simulink model "FSFB_FF_HIL_quick_dirty"  (R2022a)
settings: Solver=FixedStepAuto  StartTime=tspan(1)  StopTime=tspan(2)  FixedStep=Ts  RelTol=1e-9
undefined symbols (not defined in the file): A, B, DiscIntNeverNeededParam, H, K1, K2, Q_KF, R_KF, Serial_Port, Standard_Devices, Ts, VDefs
libraries: simulink_extras x8, sldrtlib x2, dspsigops x1
settings Model: SimulationMode=external  Creator=zachn  LastModifiedBy=domin
settings SolverCC: AlgebraicLoopSolver=TrustRegion
settings DataIOCC: SaveFormat=StructureWithTime  InspectSignalLogs=on
settings DebuggingCC: UnconnectedInputMsg=warning  UnconnectedOutputMsg=warning  UnconnectedLineMsg=warning  SFMachineParentedDataDiag=warning
settings HardwareCC: ProdBitPerLong=64  ProdHWDeviceType=Intel->x86-64 (Linux 64)
settings RTWCC: Description=Simulink Desktop Real-Time  SystemTargetFile=sldrt.tlc  TemplateMakefile=sldrt.tmf  RTWCompilerOptimization=on  DLArmComputeVersion=19.05
settings CodeAppCC: MaxIdLength=95
settings SimulinkDesktopRealTimeCC: TargetLibSuffix=_sldrt.a  TargetPreCompLibLocation=C:\Program Files\MATLAB\R2022a\toolbox\sldrt\lib\win64

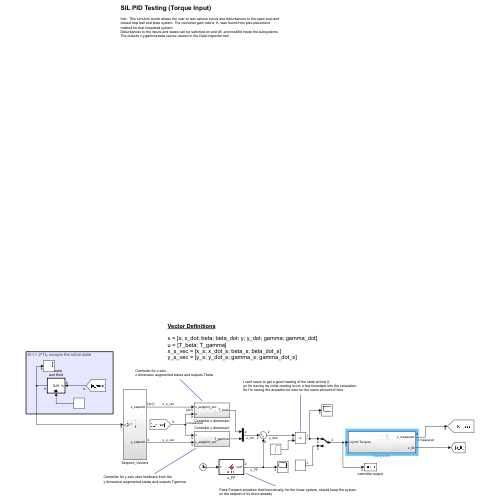
[thumbnail: Simulink's stored preview of the top-level diagram]
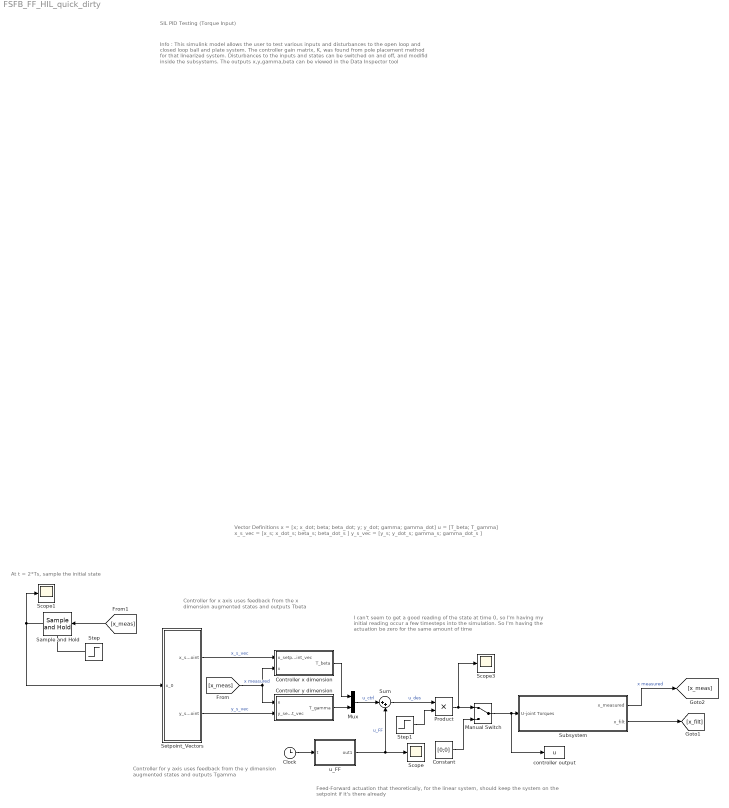
== system FSFB_FF_HIL_quick_dirty ==
  note: At t = 2*Ts, sample the initial state
  note: I can't seem to get a good reading of the state at time 0,
      | so I'm having my initial reading occur a few timesteps into the simulation.
      | So I'm having the actuation be zero for the same amount of time
  note: Info : This simulink model allows the user to test various inputs and disturbances to the open loop and closed loop ball and plate system. The controller gain matrix, K, was found from pole placement
      | method for that linearized system.
      | Disturbances to the inputs and states can be switched on and off, and modifid inside the subsystems.
      | The outputs x,y,gamma,beta can be viewed in the Data Inspector tool
  note: SIL PID Testing (Torque Input)
  note: Vector Definitions
      |
      | x = [x; x_dot; beta; beta_dot; y; y_dot; gamma; gamma_dot]
      | u = [T_beta; T_gamma]
      | x_s_vec = [x_s; x_dot_s; beta_s; beta_dot_s ]
      | y_s_vec = [y_s; y_dot_s; gamma_s; gamma_dot_s ]
  note: Feed-Forward actuation that theoretically, for the linear system, should keep the system on the setpoint if it's there already
  note: Controller for x axis uses feedback from the
      | x dimension augmented states and outputs Tbeta
  note: Controller for y axis uses feedback from the
      | y dimension augmented states and outputs Tgamma
  Clock : Clock
  Constant : Constant  Value=[0;0]
  Controller x dimension : Subsystem
  Controller y dimension : Subsystem
  Manual Switch : ManualSwitch
  Mux : Mux  Inputs=2
  Product : Product
  Sample and Hold : dspsigops/Sample and Hold  trig=Either edge  initCond=zeros(8,1)  latchinput=off
  Scope : Scope
  Scope1 : Scope
  Scope3 : Scope
  Setpoint_Vectors : Subsystem
  Step : Step  Time=2*Ts  SampleTime=0
  Step1 : Step  Time=2*Ts  SampleTime=0
  Subsystem : Subsystem
  Sum : Sum  Inputs=|++
  controller output : ToWorkspace  VariableName=u  SampleTime=-1
  u_FF : MATLAB Function  TreatAsAtomicUnit=on
  wires:
  Subsystem/1(x_measured) -> [x_meas]  "x measured"
  Clock/1 -> u_FF/1(t)
  Step/1 -> Sample and Hold/Trigger
  [x_meas] -> Controller y dimension/1(x), Controller x dimension/2(x)  "x measured"
  Setpoint_Vectors/1(x_setpoint) -> Controller x dimension/1(x_setpoint_vec)  "x_s_vec"
  Sum/1 -> Product/1  "u_des"
  Controller x dimension/1(T_beta) -> Mux/1
  Setpoint_Vectors/2(y_setpoint) -> Controller y dimension/2(y_setpoint_vec)  "y_s_vec"
  Mux/1 -> Sum/1  "u_ctrl"
  Sample and Hold/1 -> Setpoint_Vectors/1(x_0), Scope1/1
  Controller y dimension/1(T_gamma) -> Mux/2
  u_FF/1(out1) -> Sum/2, Scope/1  "u_FF"
  Subsystem/2(x_filt) -> [x_filt]
  [x_meas] -> Sample and Hold/1
  Product/1 -> Manual Switch/1, Scope3/1
  Step1/1 -> Product/2
  Manual Switch/1 -> controller output/1, Subsystem/1(U-joint Torques)
  Constant/1 -> Manual Switch/2

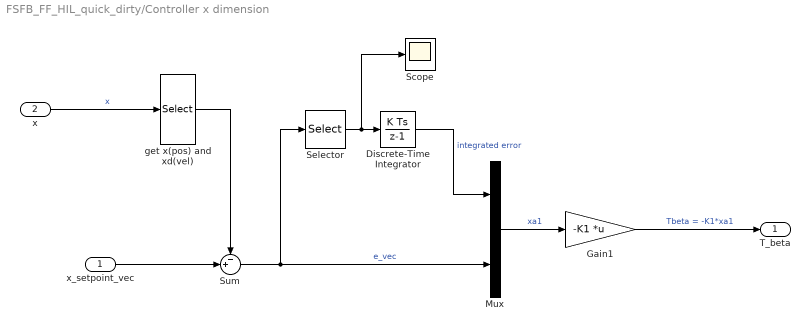
== system FSFB_FF_HIL_quick_dirty/Controller x dimension ==
  x_setpoint_vec : Inport
  x : Inport  Port=2
  Discrete-Time Integrator : DiscreteIntegrator  SampleTime=Ts  ICPrevOutput=DiscIntNeverNeededParam  ICPrevScaledInput=DiscIntNeverNeededParam
  Gain1 : Gain  Gain=-K1  Multiplication=Matrix(K*u)
  Mux : Mux  Inputs=2
  Scope : Scope
  Selector : Selector  InputPortWidth=4  IndexOptions=Index vector (dialog)  Indices=[1 ]  OutputSizes=1
  Sum : Sum  Inputs=-+|
  get x(pos) and xd(vel) : Selector  InputPortWidth=8  IndexOptions=Index vector (dialog)  Indices=[1:4]  OutputSizes=1
  T_beta : Outport
  wires:
  Gain1/1 -> T_beta/1  "Tbeta = -K1*xa1"
  get x(pos) and xd(vel)/1 -> Sum/1
  Mux/1 -> Gain1/1  "xa1"
  Sum/1 -> Selector/1, Mux/2  "e_vec"
  x_setpoint_vec/1 -> Sum/2
  x/1 -> get x(pos) and xd(vel)/1  "x"
  Selector/1 -> Discrete-Time Integrator/1, Scope/1
  Discrete-Time Integrator/1 -> Mux/1  "integrated error"

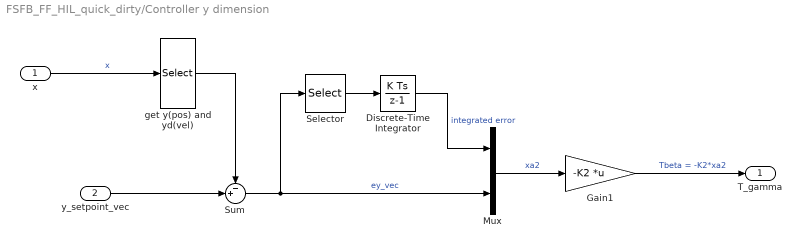
== system FSFB_FF_HIL_quick_dirty/Controller y dimension ==
  x : Inport
  y_setpoint_vec : Inport  Port=2
  Discrete-Time Integrator : DiscreteIntegrator  SampleTime=Ts  ICPrevOutput=DiscIntNeverNeededParam  ICPrevScaledInput=DiscIntNeverNeededParam
  Gain1 : Gain  Gain=-K2  Multiplication=Matrix(K*u)
  Mux : Mux  Inputs=2
  Selector : Selector  InputPortWidth=4  IndexOptions=Index vector (dialog)  Indices=[1 ]  OutputSizes=1
  Sum : Sum  Inputs=-+|
  get y(pos) and yd(vel) : Selector  InputPortWidth=8  IndexOptions=Index vector (dialog)  Indices=[5:8]  OutputSizes=1
  T_gamma : Outport
  wires:
  Discrete-Time Integrator/1 -> Mux/1  "integrated error"
  x/1 -> get y(pos) and yd(vel)/1  "x"
  Gain1/1 -> T_gamma/1  "Tbeta = -K2*xa2"
  get y(pos) and yd(vel)/1 -> Sum/1
  Mux/1 -> Gain1/1  "xa2"
  Selector/1 -> Discrete-Time Integrator/1
  Sum/1 -> Selector/1, Mux/2  "ey_vec"
  y_setpoint_vec/1 -> Sum/2

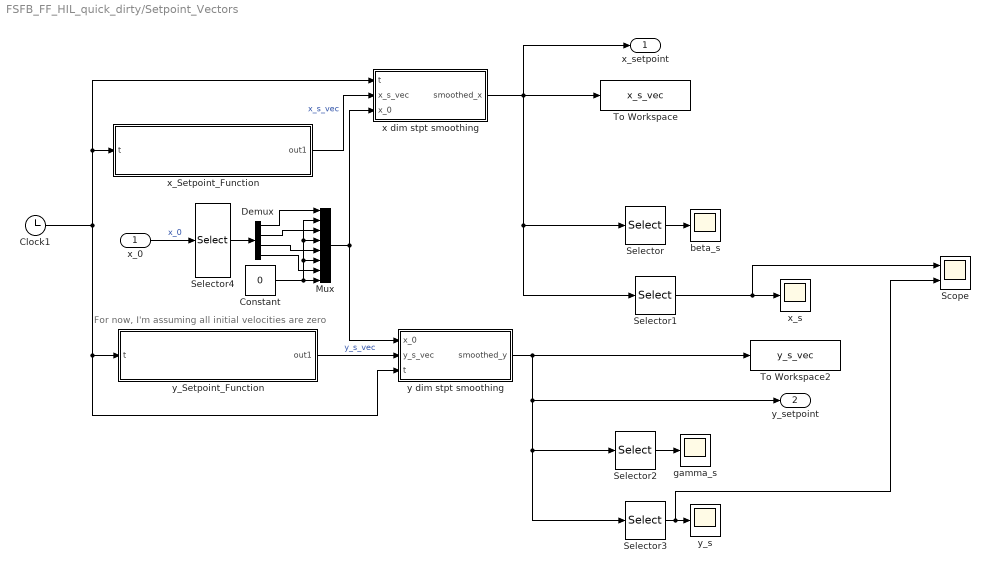
== system FSFB_FF_HIL_quick_dirty/Setpoint_Vectors ==
  note: For now, I'm assuming all initial velocities are zero
  x_0 : Inport
  Clock1 : Clock
  Constant : Constant  Value=0
  Demux : Demux
  Mux : Mux  Inputs=8
  Scope : Scope  NumInputPorts=2
  Selector : Selector  InputPortWidth=4  IndexOptions=Index vector (dialog)  Indices=[3]  OutputSizes=1
  Selector1 : Selector  InputPortWidth=4  IndexOptions=Index vector (dialog)  Indices=[1]  OutputSizes=1
  Selector2 : Selector  InputPortWidth=4  IndexOptions=Index vector (dialog)  Indices=[3]  OutputSizes=1
  Selector3 : Selector  InputPortWidth=4  IndexOptions=Index vector (dialog)  Indices=[1]  OutputSizes=1
  Selector4 : Selector  InputPortWidth=8  IndexOptions=Index vector (dialog)  Indices=[1 3 5 7]  OutputSizes=1
  To Workspace : ToWorkspace  VariableName=x_s_vec  SampleTime=-1
  To Workspace2 : ToWorkspace  VariableName=y_s_vec  SampleTime=-1
  beta_s : Scope
  gamma_s : Scope
  x dim stpt smoothing : MATLAB Function  TreatAsAtomicUnit=on
  x_Setpoint_Function : MATLAB Function  TreatAsAtomicUnit=on
  x_s : Scope
  y dim stpt smoothing : MATLAB Function  TreatAsAtomicUnit=on
  y_Setpoint_Function : MATLAB Function  TreatAsAtomicUnit=on
  y_s : Scope
  x_setpoint : Outport
  y_setpoint : Outport  Port=2
  wires:
  Clock1/1 -> y_Setpoint_Function/1(t), y dim stpt smoothing/3(t), x dim stpt smoothing/1(t), x_Setpoint_Function/1(t)
  x_Setpoint_Function/1(out1) -> x dim stpt smoothing/2(x_s_vec)  "x_s_vec"
  Selector/1 -> beta_s/1
  Selector1/1 -> Scope/1, x_s/1
  Selector3/1 -> Scope/2, y_s/1
  Selector2/1 -> gamma_s/1
  y_Setpoint_Function/1(out1) -> y dim stpt smoothing/2(y_s_vec)  "y_s_vec"
  x dim stpt smoothing/1(smoothed_x) -> Selector/1, Selector1/1, To Workspace/1, x_setpoint/1
  y dim stpt smoothing/1(smoothed_y) -> To Workspace2/1, y_setpoint/1, Selector3/1, Selector2/1
  x_0/1 -> Selector4/1  "x_0"
  Selector4/1 -> Demux/1
  Demux/1 -> Mux/1
  Mux/1 -> x dim stpt smoothing/3(x_0), y dim stpt smoothing/1(x_0)
  Constant/1 -> Mux/2, Mux/4, Mux/6, Mux/8
  Demux/4 -> Mux/7
  Demux/3 -> Mux/5
  Demux/2 -> Mux/3

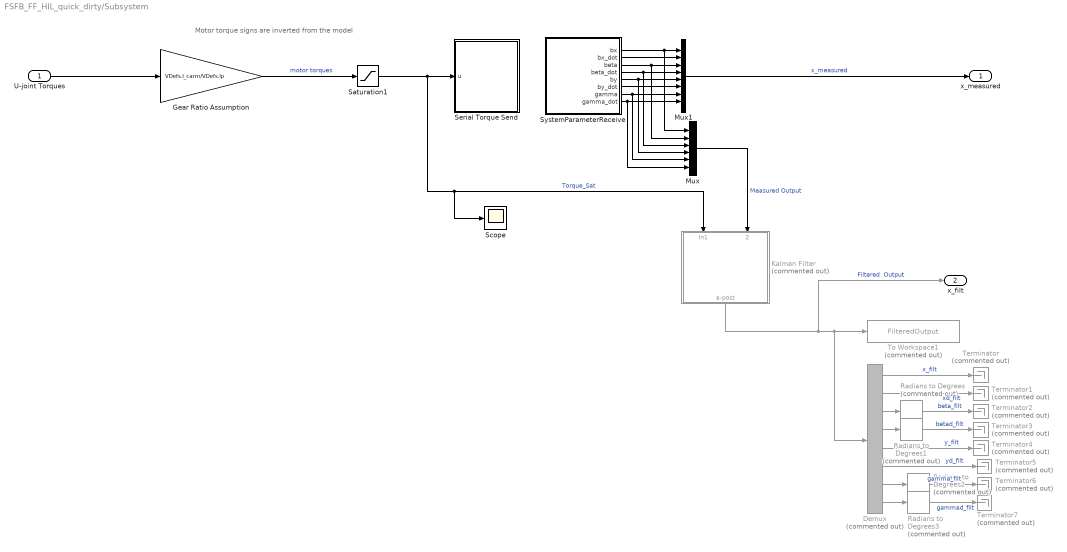
== system FSFB_FF_HIL_quick_dirty/Subsystem ==
  note: Motor torque signs are inverted from the model
  U-joint Torques : Inport
  Demux : Demux  Commented=on  Outputs=8
  Gear Ratio Assumption : Gain  Gain=VDefs.l_carm/VDefs.lp
  Kalman Filter : Subsystem  Commented=on
  Mux : Mux  Inputs=6
  Mux1 : Mux  Inputs=8
  Radians to Degrees{,1..3} (4 alike) : simulink_extras/Transformations/Radians to Degrees  Commented=on
  Saturation1 : Saturate  UpperLimit=1.5  LowerLimit=-1.5
  Scope : Scope
  Serial Torque Send : Subsystem
  SystemParameterReceive : Subsystem
  Terminator{,1..7} (8 alike) : Terminator  Commented=on
  To Workspace1 : ToWorkspace  Commented=on  VariableName=FilteredOutput  SampleTime=-1
  x_measured : Outport
  x_filt : Outport  Port=2
  wires:
  SystemParameterReceive/1(bx) -> Mux/1, Mux1/1
  SystemParameterReceive/8(gamma_dot) -> Mux/6, Mux1/8
  Gear Ratio Assumption/1 -> Saturation1/1  "motor torques"
  SystemParameterReceive/2(bx_dot) -> Mux1/2
  Saturation1/1 -> Scope/1, Kalman Filter/1(In1), Serial Torque Send/1(u)  "Torque_Sat"
  SystemParameterReceive/7(gamma) -> Mux/5, Mux1/7
  SystemParameterReceive/6(by_dot) -> Mux1/6
  SystemParameterReceive/5(by) -> Mux/4, Mux1/5
  SystemParameterReceive/4(beta_dot) -> Mux/3, Mux1/4
  SystemParameterReceive/3(beta) -> Mux/2, Mux1/3
  Mux1/1 -> x_measured/1  "x_measured"
  U-joint Torques/1 -> Gear Ratio Assumption/1
  Mux/1 -> Kalman Filter/2(Measured Output)  "Measured Output"
  Kalman Filter/1(a-post) -> x_filt/1, Demux/1, To Workspace1/1  "Filtered  Output"
  Demux/8 -> Radians to Degrees3/1
  Demux/6 -> Terminator5/1  "yd_filt"
  Demux/1 -> Terminator/1  "x_filt"
  Demux/5 -> Terminator4/1  "y_filt"
  Demux/4 -> Radians to Degrees1/1
  Demux/3 -> Radians to Degrees/1
  Demux/2 -> Terminator1/1  "xd_filt"
  Demux/7 -> Radians to Degrees2/1
  Radians to Degrees/1 -> Terminator2/1  "beta_filt"
  Radians to Degrees1/1 -> Terminator3/1  "betad_filt"
  Radians to Degrees2/1 -> Terminator6/1  "gamma_filt"
  Radians to Degrees3/1 -> Terminator7/1  "gammad_filt"

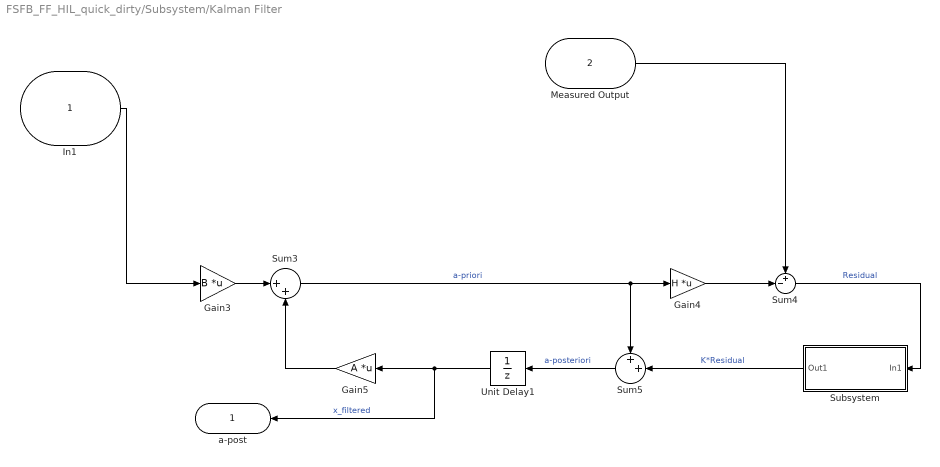
== system FSFB_FF_HIL_quick_dirty/Subsystem/Kalman Filter ==
  In1 : Inport
  Measured Output : Inport  Port=2
  Gain3 : Gain  Gain=B  Multiplication=Matrix(K*u)
  Gain4 : Gain  Gain=H  Multiplication=Matrix(K*u)
  Gain5 : Gain  Gain=A  Multiplication=Matrix(K*u)
  Subsystem : Subsystem
  Sum3 : Sum  Inputs=|++
  Sum4 : Sum  Inputs=+-|
  Sum5 : Sum  Inputs=++|
  Unit Delay1 : UnitDelay  InitialCondition=zeros(8,1)  SampleTime=Ts  HasFrameUpgradeWarning=on
  a-post : Outport  VectorParamsAs1DForOutWhenUnconnected=off
  wires:
  Unit Delay1/1 -> a-post/1, Gain5/1  "x_filtered"
  Gain4/1 -> Sum4/2
  Sum3/1 -> Sum5/1, Gain4/1  "a-priori"
  In1/1 -> Gain3/1
  Measured Output/1 -> Sum4/1
  Subsystem/1(Out1) -> Sum5/2  "K*Residual"
  Sum5/1 -> Unit Delay1/1  "a-posteriori"
  Gain5/1 -> Sum3/2
  Gain3/1 -> Sum3/1
  Sum4/1 -> Subsystem/1(In1)  "Residual"

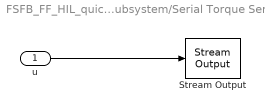
== system FSFB_FF_HIL_quick_dirty/Subsystem/Serial Torque Send ==
  u : Inport
  Stream Output : sldrtlib/Stream Output  SampleTime=Ts  MaxMissedTicks=10  ShowMissedTicks=off  YieldWhenWaiting=off  DrvName=Standard_Devices/Serial_Port  DrvAddress=6  DrvOptions=[115200 8 0 0 1 0 0 0]  PortSizes=2  FormatString='%g %g\n'  ShowReady=off  ShowError=off  InitialValue=[]  FinalValue=[]
      settings: AttributesFormatString=Serial Port [6]  SourceProductBaseCode=WT
  wires:
  u/1 -> Stream Output/1

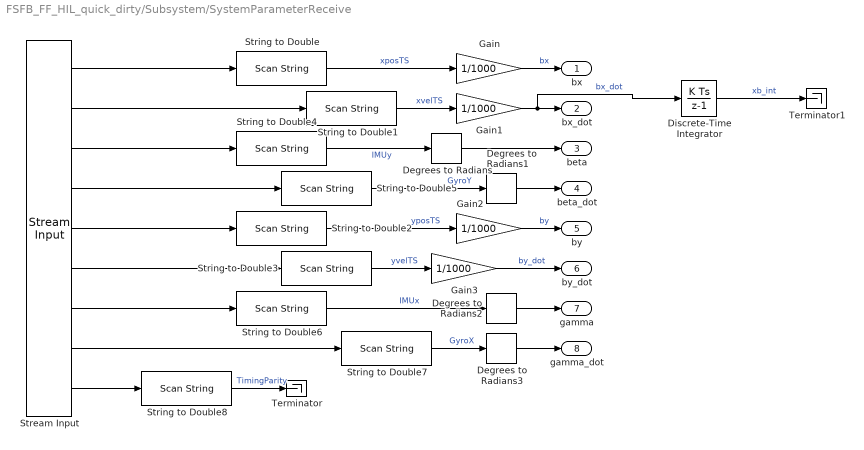
== system FSFB_FF_HIL_quick_dirty/Subsystem/SystemParameterReceive ==
  Degrees to Radians{,1..3} (4 alike) : simulink_extras/Transformations/Degrees to Radians
  Discrete-Time Integrator : DiscreteIntegrator  SampleTime=Ts  ICPrevOutput=DiscIntNeverNeededParam  ICPrevScaledInput=DiscIntNeverNeededParam
  Gain{,1..3} (4 alike) : Gain  Gain=1/1000  OutDataTypeStr=double
  Stream Input : sldrtlib/Stream Input  SampleTime=Ts  MaxMissedTicks=10  ShowMissedTicks=off  YieldWhenWaiting=on  DrvName=Standard_Devices/Serial_Port  DrvAddress=6  DrvOptions=[115200 8 0 0 1 0 0 0]  DataTypes={'string','string','string','string','string','string','string','string','string'}  FormatString='%s %s %s %s %s %s %s %s %s'  Terminator={'\r', '\n'}  ShowReady=off  ShowError=off
      settings: AttributesFormatString=Serial Port [6]  SourceProductBaseCode=WT
  String to Double : ScanString  Format="\"%d\""
  String to Double{1..8} (8 alike) : ScanString  Format="\"%lf\""
  Terminator : Terminator
  Terminator1 : Terminator
  bx : Outport
  bx_dot : Outport  Port=2
  beta : Outport  Port=3
  beta_dot : Outport  Port=4
  by : Outport  Port=5
  by_dot : Outport  Port=6
  gamma : Outport  Port=7
  gamma_dot : Outport  Port=8
  wires:
  Stream Input/1 -> String to Double/1
  Stream Input/8 -> String to Double7/1
  Degrees to Radians3/1 -> gamma_dot/1
  Degrees to Radians2/1 -> gamma/1
  Stream Input/6 -> String to Double3/1
  Stream Input/9 -> String to Double8/1
  Stream Input/5 -> String to Double2/1
  String to Double8/1 -> Terminator/1  "TimingParity"
  Stream Input/7 -> String to Double6/1
  String to Double6/1 -> Degrees to Radians2/1  "IMUx"
  Stream Input/2 -> String to Double1/1
  String to Double1/1 -> Gain1/1  "xvelTS"
  Gain1/1 -> Discrete-Time Integrator/1, bx_dot/1  "bx_dot"
  Stream Input/4 -> String to Double5/1
  Stream Input/3 -> String to Double4/1
  Gain/1 -> bx/1  "bx"
  String to Double/1 -> Gain/1  "xposTS"
  String to Double7/1 -> Degrees to Radians3/1  "GyroX"
  String to Double2/1 -> Gain2/1  "yposTS"
  Gain2/1 -> by/1  "by"
  Gain3/1 -> by_dot/1  "by_dot"
  String to Double3/1 -> Gain3/1  "yvelTS"
  Degrees to Radians1/1 -> beta_dot/1
  Degrees to Radians/1 -> beta/1
  String to Double4/1 -> Degrees to Radians/1  "IMUy"
  String to Double5/1 -> Degrees to Radians1/1  "GyroY"
  Discrete-Time Integrator/1 -> Terminator1/1  "xb_int"

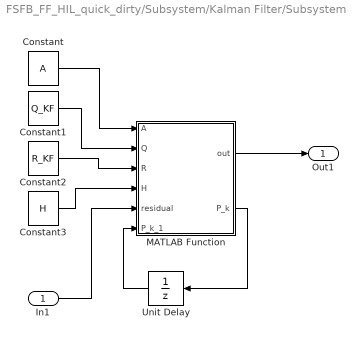
== system FSFB_FF_HIL_quick_dirty/Subsystem/Kalman Filter/Subsystem ==
  In1 : Inport
  Constant : Constant  Value=A  VectorParams1D=off
  Constant1 : Constant  Value=Q_KF  VectorParams1D=off
  Constant2 : Constant  Value=R_KF  VectorParams1D=off
  Constant3 : Constant  Value=H  VectorParams1D=off
  MATLAB Function : MATLAB Function  TreatAsAtomicUnit=on
  Unit Delay : UnitDelay  InitialCondition=zeros(8,8)  SampleTime=Ts  HasFrameUpgradeWarning=on
  Out1 : Outport  VectorParamsAs1DForOutWhenUnconnected=off
  wires:
  In1/1 -> MATLAB Function/5(residual)
  MATLAB Function/1(out) -> Out1/1
  MATLAB Function/2(P_k) -> Unit Delay/1
  Unit Delay/1 -> MATLAB Function/6(P_k_1)
  Constant/1 -> MATLAB Function/1(A)
  Constant1/1 -> MATLAB Function/2(Q)
  Constant2/1 -> MATLAB Function/3(R)
  Constant3/1 -> MATLAB Function/4(H)

== matlab function FSFB_FF_HIL_quick_dirty/Setpoint_Vectors/y dim stpt smoothing ==
  data: x_0 input size=8; y_s_vec input; t input; smoothed_y output size=4; Tau parameter
function smoothed_y = fcn(x_0,y_s_vec,t, Tau)

smoothed_y = y_s_vec*(1-exp(-t/Tau)) + x_0(5:end)*exp(-t/Tau);

== matlab function FSFB_FF_HIL_quick_dirty/Setpoint_Vectors/x_Setpoint_Function ==
  data: t input; out1 output
function out1 = x_s_vec(t)
%#codegen

%    This function was generated by the Symbolic Math Toolbox version 9.1.
%    22-Apr-2022 15:47:36

out1 = [0.0;0.0;0.0;0.0];

== matlab function FSFB_FF_HIL_quick_dirty/Setpoint_Vectors/y_Setpoint_Function ==
  data: t input; out1 output
function out1 = y_s_vec(t)
%#codegen

%    This function was generated by the Symbolic Math Toolbox version 9.1.
%    22-Apr-2022 15:47:37

out1 = [0.0;0.0;0.0;0.0];

== matlab function FSFB_FF_HIL_quick_dirty/Subsystem/Kalman Filter/Subsystem/MATLAB Function ==
  data: A input; out output size=8; Q input; R input; H input; residual input; P_k_1 input; P_k output
function [out, P_k] = fcn(A,Q,R,H,residual,P_k_1)
%Predictor
P_k_m = A*P_k_1*A' + Q;
%Corrector
K_k = P_k_m*H'/(H*P_k_m*H' + R);
P_k = (eye(size(K_k*H)) - K_k*H)*P_k_m;
out = K_k*residual;

== matlab function FSFB_FF_HIL_quick_dirty/u_FF ==
  data: out1 output size=2; t input
function out1 = u_FF(t)
%#codegen

%    This function was generated by the Symbolic Math Toolbox version 9.1.
%    22-Apr-2022 15:47:37

out1 = [0.0;0.0];

== matlab function FSFB_FF_HIL_quick_dirty/Setpoint_Vectors/x dim stpt smoothing ==
  data: t input; x_s_vec input size=4; smoothed_x output; Tau parameter; x_0 input
function smoothed_x = fcn(t,x_s_vec, Tau, x_0)

smoothed_x = x_s_vec*(1-exp(-t/Tau)) + x_0(1:4)*exp(-t/Tau);
